simulink model "DistanceMessurement"  (Simulink 6.3)
settings: Solver=VariableStepDiscrete  StartTime=0.0  StopTime=10.0  RelTol=1e-3
settings Model: LastModifiedBy=Huang

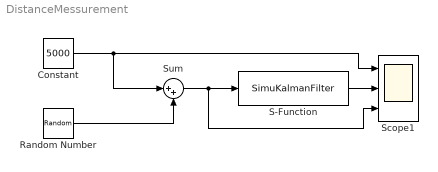
== system DistanceMessurement ==
  Constant : Constant  Value=5000  SampleTime=0.1
  Random Number : RandomNumber  Variance=5  SampleTime=0.1
  S-Function : S-Function  FunctionName=SimuKalmanFilter
  Scope1 : Scope  NumInputPorts=3
      settings: TickLabels=on  TimeRange=10  YMin=4995~4995~4995  YMax=5005~5005~5005
  Sum : Sum  Inputs=|++
  wires:
  Random Number/1 -> Sum/2
  Constant/1 -> Sum/1, Scope1/1
  Sum/1 -> S-Function/1, Scope1/3
  S-Function/1 -> Scope1/2
